simulink model "HydraulicCrane_cosim"  (R2019a)
settings: Solver=VariableStepAuto  StartTime=0.0  StopTime=20.0  RelTol=1e-3
libraries: simulink x1
settings Model: Creator=udarn  LastModifiedBy=udarn

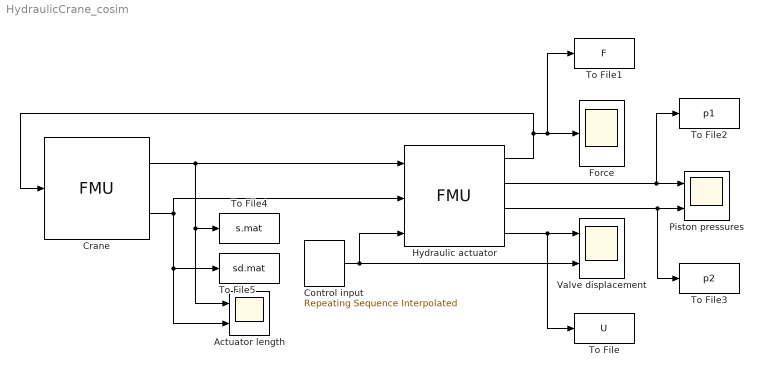
== system HydraulicCrane_cosim ==
  Actuator length : Scope  NumInputPorts=2
  Control input : simulink/Sources/Repeating Sequence Interpolated  OutValues=[0 0 0.6 0.6 -1 0 ].'  TimeValues=[0 0.5 2 7 9 10].'  LookUpMeth=Interpolation-Use End Values  tsamp=5e-4  OutMin=[]  OutMax=[]  OutDataTypeStr=double  OutputDataTypeScalingMode=double  OutDataType=fixdt(0,8)  OutScaling=2^-10
  Crane : FMU  FMUName=FMU2cs_crane.fmu  FMUMode=CoSimulation  crane_mass=500.000000  crane_length=1.000000  pend_mass=100.000000  pend_length=0.300000  crane_angle=0.523599  mask(FMU2cs_crane [Co-Simulation, v2.0]){}
      mask Display:
      | disp('FMU2cs_crane');
      | port_label('output',1,'s');
      | port_label('output',2,'sd');
      | port_label('input',1,'F');
  Force : Scope
  Hydraulic actuator : FMU  FMUName=FMU2cs_actuator.fmu  FMUMode=CoSimulation  init_F=0.000000  mask(FMU2cs_actuator [Co-Simulation, v2.0]){}
      mask Display:
      | disp('FMU2cs_actuator');
      | port_label('output',1,'F');
      | port_label('output',2,'p1');
      | port_label('output',3,'p2');
      | port_label('output',4,'U');
      | port_label('input',1,'s');
      | port_label('input',2,'sd');
      | port_label('input',3,'Uref');
  Piston pressures : Scope  NumInputPorts=2
  To File : ToFile  Filename=U  SaveFormat=Timeseries  SampleTime=1e-3
  To File1 : ToFile  Filename=F  SaveFormat=Timeseries  SampleTime=1e-3
  To File2 : ToFile  Filename=p1  SaveFormat=Timeseries  SampleTime=1e-3
  To File3 : ToFile  Filename=p2  SaveFormat=Timeseries  SampleTime=1e-3
  To File4 : ToFile  Filename=s.mat  SaveFormat=Timeseries  SampleTime=1e-3
  To File5 : ToFile  Filename=sd.mat  SaveFormat=Timeseries  SampleTime=1e-3
  Valve displacement : Scope  NumInputPorts=2
  wires:
  Crane/1 -> Actuator length/1, To File4/1, Hydraulic actuator/1
  Crane/2 -> Hydraulic actuator/2, To File5/1, Actuator length/2
  Control input/1 -> Valve displacement/2, Hydraulic actuator/3
  Hydraulic actuator/1 -> Crane/1, To File1/1, Force/1
  Hydraulic actuator/2 -> To File2/1, Piston pressures/1
  Hydraulic actuator/3 -> To File3/1, Piston pressures/2
  Hydraulic actuator/4 -> To File/1, Valve displacement/1
